simulink subsystem "Reverse_Propulsion_Model"  (R2023b)
settings: Solver=VariableStepAuto  StartTime=0.0  StopTime=10.0  RelTol=1e-3
undefined symbols (not defined in the file): dataBase
settings Model: Creator=cyber  LastModifiedBy=cyber

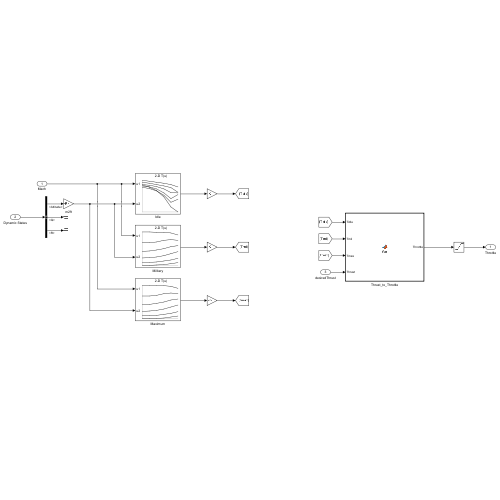
[thumbnail: Simulink's stored preview of the top-level diagram]
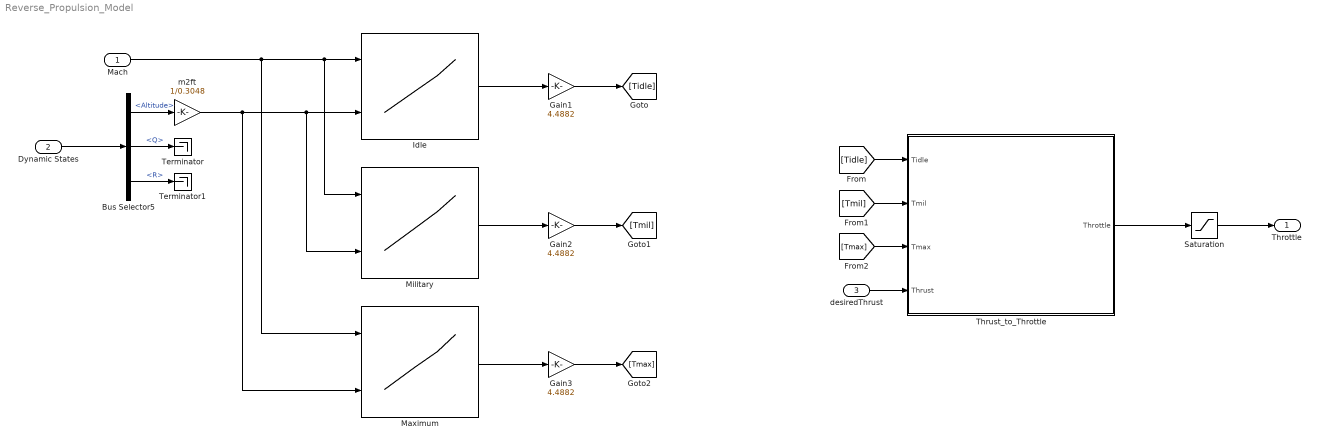
== system Reverse_Propulsion_Model ==
  Mach : Inport
  Dynamic States : Inport  Port=2
  desiredThrust : Inport  Port=3
  Bus Selector5 : BusSelector  OutputSignals=Altitude,Q,R
  Gain1 : Gain  Gain=4.4882
  Gain2 : Gain  Gain=4.4882
  Gain3 : Gain  Gain=4.4882
  Idle : Lookup_n-D  BreakpointsForDimension1=dataBase.Engine.f16_EngineData.BP.idle.mach  BreakpointsForDimension2=dataBase.Engine.f16_EngineData.BP.idle.alt_ft  BeginIndexSearchUsingPreviousIndexResult=on  Table=dataBase.Engine.f16_EngineData.data.Thrust_lbs.idle  ExtrapMethod=Clip  InternalRulePriority=Speed  RndMeth=Simplest
      settings: InputPortMap=u0,u1
  Maximum : Lookup_n-D  BreakpointsForDimension1=dataBase.Engine.f16_EngineData.BP.mil.mach  BreakpointsForDimension2=dataBase.Engine.f16_EngineData.BP.mil.alt_ft  BeginIndexSearchUsingPreviousIndexResult=on  Table=dataBase.Engine.f16_EngineData.data.Thrust_lbs.mil  ExtrapMethod=Clip  InternalRulePriority=Speed  RndMeth=Simplest
      settings: InputPortMap=u0,u1
  Military : Lookup_n-D  BreakpointsForDimension1=dataBase.Engine.f16_EngineData.BP.mil.mach  BreakpointsForDimension2=dataBase.Engine.f16_EngineData.BP.mil.alt_ft  BeginIndexSearchUsingPreviousIndexResult=on  Table=dataBase.Engine.f16_EngineData.data.Thrust_lbs.mil  ExtrapMethod=Clip  InternalRulePriority=Speed  RndMeth=Simplest
      settings: InputPortMap=u0,u1
  Saturation : Saturate  UpperLimit=100  LowerLimit=0
  Terminator : Terminator
  Terminator1 : Terminator
  Thrust_to_Throttle : MATLAB Function  TreatAsAtomicUnit=on
  m2ft : Gain  Gain=1/0.3048
  Throttle : Outport
  wires:
  desiredThrust/1 -> Thrust_to_Throttle/4(Thrust)
  Thrust_to_Throttle/1(Throttle) -> Saturation/1
  Bus Selector5/3 -> Terminator1/1  "<R>"
  Bus Selector5/2 -> Terminator/1  "<Q>"
  Dynamic States/1 -> Bus Selector5/1
  Bus Selector5/1 -> m2ft/1  "<Altitude>"
  Mach/1 -> Maximum/1, Military/1, Idle/1
  Gain2/1 -> [Tmil]
  m2ft/1 -> Maximum/2, Military/2, Idle/2
  [Tmax] -> Thrust_to_Throttle/3(Tmax)
  Military/1 -> Gain2/1
  Maximum/1 -> Gain3/1
  Gain1/1 -> [Tidle]
  Idle/1 -> Gain1/1
  Gain3/1 -> [Tmax]
  [Tmil] -> Thrust_to_Throttle/2(Tmil)
  [Tidle] -> Thrust_to_Throttle/1(Tidle)
  Saturation/1 -> Throttle/1

== matlab function Reverse_Propulsion_Model/Thrust_to_Throttle ==
  data: Tidle input size=1; Throttle output size=1; Tmil input size=1; Tmax input size=1; Thrust input size=1
function Throttle = fcn(Tidle, Tmil, Tmax, Thrust)
Pc_lt_50 = (Thrust -Tidle)*50/(Tmil - Tidle);  %lt: less than
Pc_ge_50 = (Thrust-Tmil)*50 /(Tmax - Tmil)+50; %ge: great equal


if Pc_lt_50 < 50
    Pc = Pc_lt_50;
elseif 50 <= Pc_ge_50
    Pc = Pc_ge_50;
else
    Pc = Pc_lt_50;
end


Throttle_le_77 = Pc*100/64.94;          % le: less equal
Throttle_gt_77 = 100*(Pc+117.38)/217.38; % gt: greater than

if Throttle_le_77 <= 77
    Throttle = Throttle_le_77 ;
elseif Throttle_gt_77 > 77
    Throttle = Throttle_gt_77;
else
    Throttle = Throttle_le_77;
end

Throttle(Throttle>100) = 100;
Throttle(Throttle<0) = 0;
